simulink library "pv_cost"  (R2025b)
settings: Solver=VariableStepAuto  StartTime=0.0  StopTime=10.0  RelTol=1e-3
settings Model: Creator=ciepm  LastModifiedBy=charlielenk

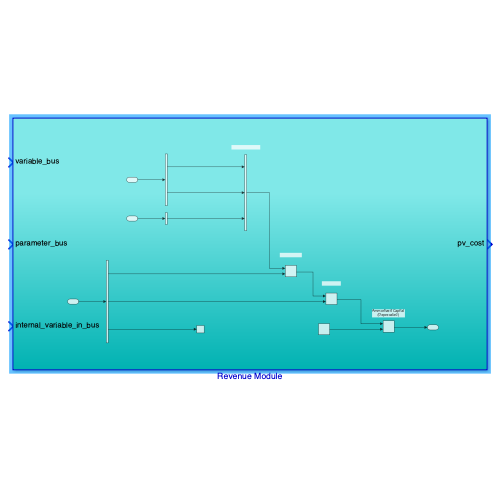
[thumbnail: Simulink's stored preview of the top-level diagram]
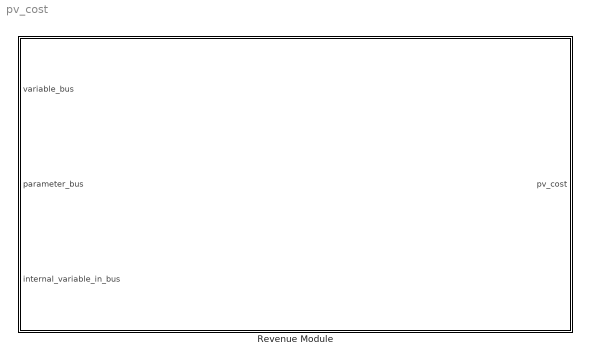
== system pv_cost ==
  Revenue Module : Subsystem

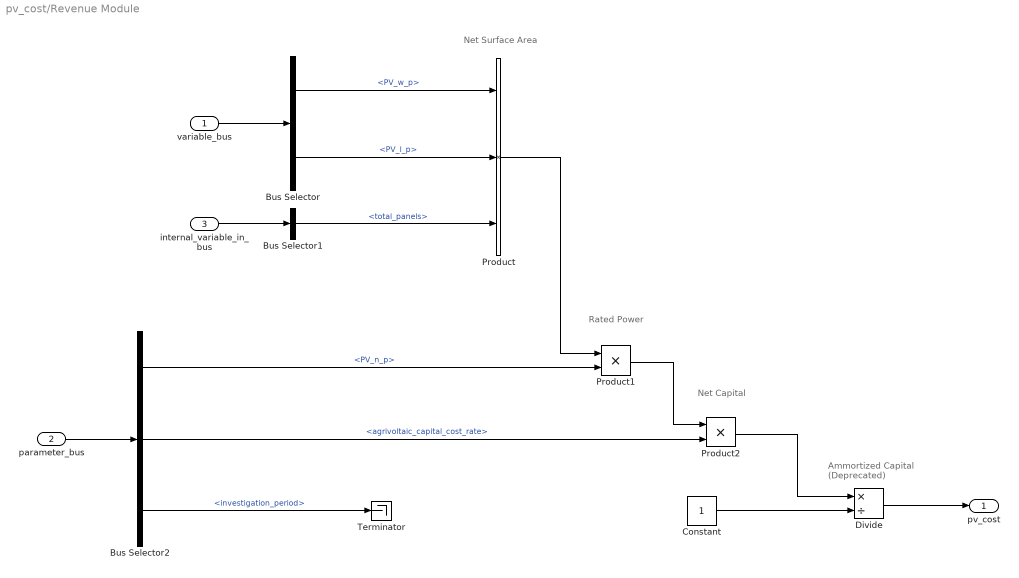
== system pv_cost/Revenue Module ==
  note: Net Surface Area
  note: Rated Power
  note: Net Capital
  note: Ammortized Capital
      | (Deprecated)
  variable_bus : Inport
  parameter_bus : Inport  Port=2
  internal_variable_in_bus : Inport  Port=3
  Bus Selector : BusSelector  OutputSignals=PV_w_p,PV_l_p
  Bus Selector1 : BusSelector  OutputSignals=energy_per_year.total_panels
  Bus Selector2 : BusSelector  OutputSignals=PV_n_p,agrivoltaic_capital_cost_rate,investigation_period
  Constant : Constant
  Divide : Product  Inputs=*/
  Product : Product  Inputs=3
  Product1 : Product
  Product2 : Product
  Terminator : Terminator
  pv_cost : Outport
  wires:
  Constant/1 -> Divide/2
  Product2/1 -> Divide/1
  Product1/1 -> Product2/1
  Bus Selector2/2 -> Product2/2  "<agrivoltaic_capital_cost_rate>"
  Product/1 -> Product1/1
  Divide/1 -> pv_cost/1
  Bus Selector/2 -> Product/2  "<PV_l_p>"
  Bus Selector/1 -> Product/1  "<PV_w_p>"
  Bus Selector2/3 -> Terminator/1  "<investigation_period>"
  Bus Selector1/1 -> Product/3  "<total_panels>"
  Bus Selector2/1 -> Product1/2  "<PV_n_p>"
  internal_variable_in_bus/1 -> Bus Selector1/1
  parameter_bus/1 -> Bus Selector2/1
  variable_bus/1 -> Bus Selector/1
